simulink model "can8auto"  (R2018a)
settings: Solver=VariableStepAuto  StartTime=0.0  StopTime=5000  RelTol=1e-3
libraries: commcrc2 x20, simulink x20, simulink_extras x5, dspswit3 x5
(part 2 of 7)

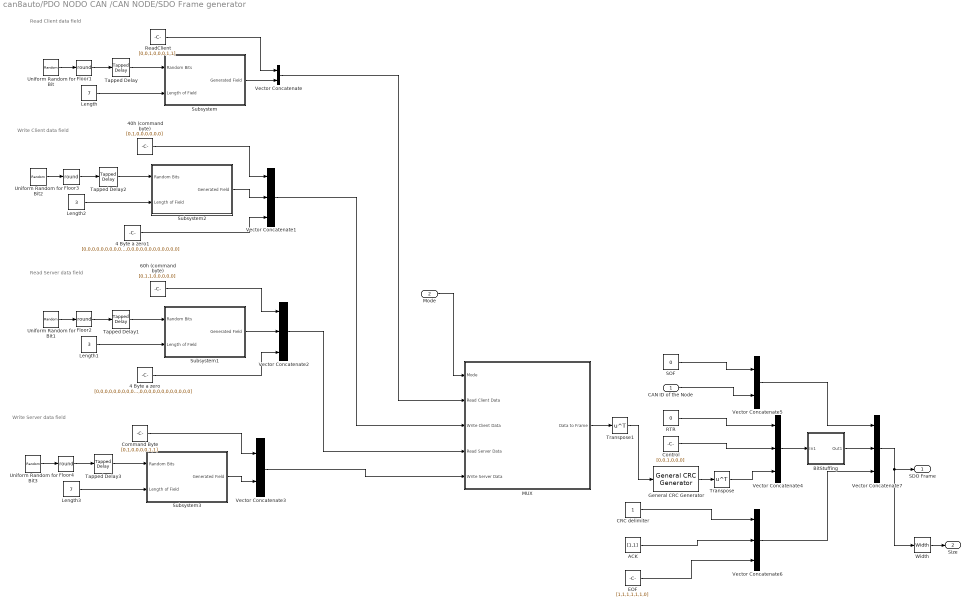
== system can8auto/PDO NODO CAN /CAN NODE/SDO Frame generator ==
  note: Read Server data field
  note: Read Client data field
  note: Write Client data field
  note: Write Server data field
  CAN ID of the Node : Inport
  Mode : Inport  Port=2
  4 Byte a zero : Constant  Value=[0,0,0,0,0,0,0,0,0,0,0,0,0,0,0,0,0,0,0,0,0,0,0,0,0,0,0,0,0,0,0,0]  VectorParams1D=off
  4 Byte a zero1 : Constant  Value=[0,0,0,0,0,0,0,0,0,0,0,0,0,0,0,0,0,0,0,0,0,0,0,0,0,0,0,0,0,0,0,0]  VectorParams1D=off
  40h (command byte) : Constant  Value=[0,1,0,0,0,0,0,0]  VectorParams1D=off
  60h (command byte) : Constant  Value=[0,1,1,0,0,0,0,0]  VectorParams1D=off
  ACK : Constant  Value=[1,1]  VectorParams1D=off
  BitStuffing : Subsystem
  CRC delimiter : Constant  VectorParams1D=off
  Command Byte : Constant  Value=[0,1,0,0,0,0,1,1]  VectorParams1D=off
  Control : Constant  Value=[0,0,1,0,0,0]  VectorParams1D=off
  EOF : Constant  Value=[1,1,1,1,1,1,0]  VectorParams1D=off
  Floor{1..4} (4 alike) : Rounding  Operator=round
  General CRC Generator : commcrc2/General CRC Generator  genPoly='z^15 + z^14 + z^10 + z^8 + z^7 + z^4 + z^3 + 1'  iniStates=0  directMethod=off  reflectInputBytes=off  reflectChecksums=off  finalXOR=0  numChecksums=1
      settings: SourceProductName=Communications Toolbox  SourceProductBaseCode=CM
  Length : Constant  Value=7  VectorParams1D=off
  Length1 : Constant  Value=3  VectorParams1D=off
  Length2 : Constant  Value=3  VectorParams1D=off
  Length3 : Constant  Value=7  VectorParams1D=off
  MUX : Subsystem
  RTR : Constant  Value=0  VectorParams1D=off
  ReadClient : Constant  Value=[0,0,1,0,0,0,1,1]  VectorParams1D=off
  SOF : Constant  Value=0  VectorParams1D=off
  Subsystem : Subsystem
  Subsystem1 : Subsystem
  Subsystem2 : Subsystem
  Subsystem3 : Subsystem
  Tapped Delay{,1..3} (4 alike) : simulink/Discrete/Tapped Delay  vinit=0  samptime=-1  NumDelays=8*8  DelayOrder=Oldest  includeCurrent=off
  Transpose : Math  Operator=transpose  SaturateOnIntegerOverflow=on
  Transpose1 : Math  Operator=transpose  SaturateOnIntegerOverflow=on
  Uniform Random for Bit{,1..3} (4 alike) : UniformRandomNumber  Minimum=0  SampleTime=0.01
  Vector Concatenate : Concatenate
  Vector Concatenate{1..2,4,6..7} (5 alike) : Concatenate  NumInputs=3
  Vector Concatenate3 : Concatenate
  Vector Concatenate5 : Concatenate
  Width : Width
  SDO Frame : Outport
  " Size" : Outport  Port=2
  wires:
  Vector Concatenate7/1 -> SDO Frame/1, Width/1
  Vector Concatenate5/1 -> Vector Concatenate7/1
  Vector Concatenate6/1 -> Vector Concatenate7/3
  BitStuffing/1(Out1) -> Vector Concatenate7/2
  Vector Concatenate4/1 -> BitStuffing/1(In1)
  RTR/1 -> Vector Concatenate4/1
  CRC delimiter/1 -> Vector Concatenate6/1
  ACK/1 -> Vector Concatenate6/2
  EOF/1 -> Vector Concatenate6/3
  CAN ID of the Node/1 -> Vector Concatenate5/2
  SOF/1 -> Vector Concatenate5/1
  MUX/1(Data to Frame) -> Transpose1/1
  Vector Concatenate3/1 -> MUX/5(Write Server Data)
  Vector Concatenate2/1 -> MUX/4(Read Server Data)
  Mode/1 -> MUX/1(Mode)
  Vector Concatenate1/1 -> MUX/3(Write Client Data)
  Vector Concatenate/1 -> MUX/2(Read Client Data)
  Width/1 -> " Size"/1
  ReadClient/1 -> Vector Concatenate/1
  Floor2/1 -> Tapped Delay1/1
  Subsystem/1(Generated Field) -> Vector Concatenate/2
  General CRC Generator/1 -> Transpose/1
  Length3/1 -> Subsystem3/2(Length of Field)
  Transpose/1 -> Vector Concatenate4/3
  4 Byte a zero/1 -> Vector Concatenate2/3
  4 Byte a zero1/1 -> Vector Concatenate1/3
  Control/1 -> Vector Concatenate4/2
  Subsystem2/1(Generated Field) -> Vector Concatenate1/2
  Tapped Delay1/1 -> Subsystem1/1(Random Bits)
  Floor1/1 -> Tapped Delay/1
  Uniform Random for Bit2/1 -> Floor3/1
  Subsystem1/1(Generated Field) -> Vector Concatenate2/2
  Subsystem3/1(Generated Field) -> Vector Concatenate3/2
  Command Byte/1 -> Vector Concatenate3/1
  Tapped Delay3/1 -> Subsystem3/1(Random Bits)
  Floor4/1 -> Tapped Delay3/1
  40h (command byte)/1 -> Vector Concatenate1/1
  Length2/1 -> Subsystem2/2(Length of Field)
  Uniform Random for Bit1/1 -> Floor2/1
  Length/1 -> Subsystem/2(Length of Field)
  Uniform Random for Bit3/1 -> Floor4/1
  Length1/1 -> Subsystem1/2(Length of Field)
  Tapped Delay/1 -> Subsystem/1(Random Bits)
  Floor3/1 -> Tapped Delay2/1
  Uniform Random for Bit/1 -> Floor1/1
  60h (command byte)/1 -> Vector Concatenate2/1
  Transpose1/1 -> General CRC Generator/1
  Tapped Delay2/1 -> Subsystem2/1(Random Bits)

== system can8auto/PDO NODO CAN /CAN NODE/SYNC Frame Generator ==
  ACK : Constant  Value=[1,1]  VectorParams1D=off
  BitStuffing : Subsystem
  COB ID (080h) : Constant  Value=[0,0,0,1,0,0,0,0,0,0,0]  VectorParams1D=off
  CRC delimiter : Constant  VectorParams1D=off
  Control : Constant  Value=[0,0,0,0,0,1]  VectorParams1D=off
  Data : Constant  Value=[0,0,0,0,0,0,0,0]'  VectorParams1D=off
  EOF : Constant  Value=[1,1,1,1,1,1,0]  VectorParams1D=off
  General CRC Generator : commcrc2/General CRC Generator  genPoly='z^15 + z^14 + z^10 + z^8 + z^7 + z^4 + z^3 + 1'  iniStates=0  directMethod=off  reflectInputBytes=off  reflectChecksums=off  finalXOR=0  numChecksums=1
      settings: SourceProductName=Communications Toolbox  SourceProductBaseCode=CM
  Mux1 : Mux  Inputs=3
  Mux2 : Mux  Inputs=2
  Mux3 : Mux  Inputs=3
  Mux4 : Mux  Inputs=3
  RTR : Constant  Value=0  VectorParams1D=off
  SOF : Constant  Value=0  VectorParams1D=off
  Transpose : Math  Operator=transpose  SaturateOnIntegerOverflow=on
  Width : Width
  SYNC Frame : Outport
  " Size" : Outport  Port=2
  wires:
  Mux4/1 -> SYNC Frame/1, Width/1
  Mux1/1 -> Mux4/1
  Mux2/1 -> Mux4/3
  BitStuffing/1(Out1) -> Mux4/2
  Mux3/1 -> BitStuffing/1(In1)
  Width/1 -> " Size"/1
  CRC delimiter/1 -> Mux3/3
  EOF/1 -> Mux2/2
  ACK/1 -> Mux2/1
  COB ID (080h)/1 -> Mux1/2
  SOF/1 -> Mux1/1
  Control/1 -> Mux3/1
  General CRC Generator/1 -> Transpose/1
  Transpose/1 -> Mux3/2
  RTR/1 -> Mux1/3
  Data/1 -> General CRC Generator/1

== system can8auto/PDO NODO CAN /CAN NODE/Triggered Subsystem1 ==
  In1 : Inport
  Trigger : TriggerPort  VariantControl=Variant
  Out1 : Outport  InitialOutput=[1,1,1,1,1,1,1,1,1,1,1,1,1,1,1,1,1,1,1,1,1,1,1,1,1,1,1,1,1,1,1,1,1,1,1,1,1,1,1,1,1,1,1,1,1,1,1,1,1,1,1,1,1,1,1,1,1,1,1,1,1,1,1,1,1,1,1,1,1,1,1,1,1,1,1,1,1,1,1,1,1,1,1,1]
  wires:
  In1/1 -> Out1/1

== system can8auto/PDO NODO CAN /Start on push/Start on push ==
  In1 : Inport
  Trigger : TriggerPort  VariantControl=Variant
  Out1 : Outport  InitialOutput=[0]
  wires:
  In1/1 -> Out1/1

== system can8auto/SDO NODO CAN/CAN NODE/Bootup Frame generator ==
  note: CAN ID / COB ID
  ID of the Node : Inport
  11-bit Adder : Subsystem
  700h : Constant  Value=[1,1,1,0,0,0,0,0,0,0,0]  VectorParams1D=off
  ACK : Constant  Value=[1,1]  VectorParams1D=off
  BitStuffing : Subsystem
  CRC delimiter : Constant  VectorParams1D=off
  Control : Constant  Value=[0,0,0,0,0,1]  VectorParams1D=off
  "Data (Bootup State) " : Constant  Value=[0,0,0,0,0,0,0,0]'  VectorParams1D=off
  EOF : Constant  Value=[1,1,1,1,1,1,0]  VectorParams1D=off
  General CRC Generator : commcrc2/General CRC Generator  genPoly='z^15 + z^14 + z^10 + z^8 + z^7 + z^4 + z^3 + 1'  iniStates=0  directMethod=off  reflectInputBytes=off  reflectChecksums=off  finalXOR=0  numChecksums=1
      settings: SourceProductName=Communications Toolbox  SourceProductBaseCode=CM
  Mux : Mux  Inputs=3
  Mux1 : Mux  Inputs=2
  Mux2 : Mux  Inputs=3
  Mux3 : Mux  Inputs=3
  RTR : Constant  Value=0  VectorParams1D=off
  SOF : Constant  Value=0  VectorParams1D=off
  Transpose : Math  Operator=transpose  SaturateOnIntegerOverflow=on
  Width : Width
  Bootload Frame : Outport
  " Size" : Outport  Port=2
  wires:
  Mux1/1 -> Mux3/1
  Mux2/1 -> Mux3/3
  BitStuffing/1(Out1) -> Mux3/2
  Mux3/1 -> Bootload Frame/1, Width/1
  Transpose/1 -> Mux/3
  RTR/1 -> Mux/1
  EOF/1 -> Mux2/3
  ACK/1 -> Mux2/2
  CRC delimiter/1 -> Mux2/1
  SOF/1 -> Mux1/1
  11-bit Adder/1(Out1) -> Mux1/2
  Width/1 -> " Size"/1
  ID of the Node/1 -> 11-bit Adder/2(In2)
  700h/1 -> 11-bit Adder/1(In1)
  Control/1 -> Mux/2
  "Data (Bootup State) "/1 -> General CRC Generator/1
  General CRC Generator/1 -> Transpose/1
  Mux/1 -> BitStuffing/1(In1)

== system can8auto/SDO NODO CAN/CAN NODE/Frame MUX ==
  Frame Kind : Inport
  Bootload Frame : Inport  Port=2
  Size Bootload : Inport  Port=3
  NMT Frame : Inport  Port=4
  Size NMT : Inport  Port=5
  SDO Frame : Inport  Port=6
  Size SDO : Inport  Port=7
  PDO Frame : Inport  Port=8
  Size PDO : Inport  Port=9
  SYNC Frame : Inport  Port=10
  Size SYNC : Inport  Port=11
  MATLAB Function2 : MATLAB Function  TreatAsAtomicUnit=on
  Vector Concatenate : Concatenate  NumInputs=5
  Vector Concatenate1 : Concatenate  NumInputs=5
  Frame to Send : Outport
  wires:
  Vector Concatenate1/1 -> MATLAB Function2/3(size)
  SYNC Frame/1 -> Vector Concatenate/5
  Size NMT/1 -> Vector Concatenate1/2
  Size SDO/1 -> Vector Concatenate1/3
  Size Bootload/1 -> Vector Concatenate1/1
  Size SYNC/1 -> Vector Concatenate1/5
  Vector Concatenate/1 -> MATLAB Function2/2(u1)
  SDO Frame/1 -> Vector Concatenate/3
  MATLAB Function2/1(result) -> Frame to Send/1
  Bootload Frame/1 -> Vector Concatenate/1
  PDO Frame/1 -> Vector Concatenate/4
  Frame Kind/1 -> MATLAB Function2/1(mode)
  NMT Frame/1 -> Vector Concatenate/2
  Size PDO/1 -> Vector Concatenate1/4

== system can8auto/SDO NODO CAN/CAN NODE/NMT Frame generator ==
  note: DATA FIELD
  Address node : Inport
  11-bit Adder : Subsystem
  ACK : Constant  Value=[1,1]  VectorParams1D=off
  BitStuffing : Subsystem
  COB ID : Constant  Value=[0,0,0,0,0,0,0,0,0,0,0]  VectorParams1D=off
  CRC delimiter : Constant  VectorParams1D=off
  Control : Constant  Value=[0,0,0,0,1,0]  VectorParams1D=off
  DATA (part1) : Constant  Value=[0,0,0,0,0]  VectorParams1D=off
  "Data " : Constant  Value=[0,0,1,0,0,0,0,0,0,0,0]  VectorParams1D=off
  EOF : Constant  Value=[1,1,1,1,1,1,0]  VectorParams1D=off
  General CRC Generator : commcrc2/General CRC Generator  genPoly='z^15 + z^14 + z^10 + z^8 + z^7 + z^4 + z^3 + 1'  iniStates=0  directMethod=off  reflectInputBytes=off  reflectChecksums=off  finalXOR=0  numChecksums=1
      settings: SourceProductName=Communications Toolbox  SourceProductBaseCode=CM
  Mux : Mux  Inputs=3
  Mux1 : Mux  Inputs=2
  Mux2 : Mux  Inputs=2
  Mux3 : Mux  Inputs=3
  Mux4 : Mux  Inputs=3
  RTR : Constant  Value=0  VectorParams1D=off
  SOF : Constant  Value=0  VectorParams1D=off
  Transpose : Math  Operator=transpose  SaturateOnIntegerOverflow=on
  Transpose1 : Math  Operator=transpose  SaturateOnIntegerOverflow=on
  Width : Width
  NMT Frame : Outport
  " Size" : Outport  Port=2
  wires:
  Mux4/1 -> Width/1, NMT Frame/1
  Mux3/1 -> Mux4/3
  Mux2/1 -> Mux4/1
  BitStuffing/1(Out1) -> Mux4/2
  Mux/1 -> BitStuffing/1(In1)
  RTR/1 -> Mux/1
  CRC delimiter/1 -> Mux3/1
  ACK/1 -> Mux3/2
  EOF/1 -> Mux3/3
  SOF/1 -> Mux2/1
  COB ID/1 -> Mux2/2
  Width/1 -> " Size"/1
  Transpose1/1 -> General CRC Generator/1
  Mux1/1 -> Transpose1/1
  11-bit Adder/1(Out1) -> Mux1/2
  DATA (part1)/1 -> Mux1/1
  "Data "/1 -> 11-bit Adder/1(In1)
  Address node/1 -> 11-bit Adder/2(In2)
  Transpose/1 -> Mux/3
  Control/1 -> Mux/2
  General CRC Generator/1 -> Transpose/1

== system can8auto/SDO NODO CAN/CAN NODE/PDO Frame Generator ==
  note: PDO DATA field
  note: CONTROL field
  CAN ID : Inport
  Data Length : Inport  Port=2
  " default = 8" : SwitchCase  CaseConditions={2,4}
  2 byte : Constant  Value=[0,0,0,0,1,0]  VectorParams1D=off
  4 byte : Constant  Value=[0,0,0,1,0,0]  VectorParams1D=off
  8 byte : Constant  Value=[0,0,1,0,0,0]  VectorParams1D=off
  ACK : Constant  Value=[1,1]  VectorParams1D=off
  CRC delimiter : Constant  VectorParams1D=off
  EOF : Constant  Value=[1,1,1,1,1,1,0]  VectorParams1D=off
  Floor1 : Rounding  Operator=round
  General CRC Generator : commcrc2/General CRC Generator  genPoly='z^15 + z^14 + z^10 + z^8 + z^7 + z^4 + z^3 + 1'  iniStates=0  directMethod=off  reflectInputBytes=off  reflectChecksums=off  finalXOR=0  numChecksums=1
      settings: SourceProductName=Communications Toolbox  SourceProductBaseCode=CM
  Merge1 : Merge  Inputs=3
  RTR : Constant  Value=0  VectorParams1D=off
  SOF : Constant  Value=0  VectorParams1D=off
  Subsystem : Subsystem
  Switch Case Action Subsystem : Subsystem  TreatAsAtomicUnit=on
  Switch Case Action Subsystem1 : Subsystem  TreatAsAtomicUnit=on
  Switch Case Action Subsystem2 : Subsystem  TreatAsAtomicUnit=on
  Tapped Delay : simulink/Discrete/Tapped Delay  vinit=0  samptime=-1  NumDelays=8*8  DelayOrder=Oldest  includeCurrent=off
  Uniform Random for Bit : UniformRandomNumber  Minimum=0  SampleTime=0.01
  Vector Concatenate1 : Concatenate  NumInputs=8
  Width : Width
  PDO Frame : Outport
  " Size" : Outport  Port=2
  wires:
  Vector Concatenate1/1 -> PDO Frame/1, Width/1
  Width/1 -> " Size"/1
  ACK/1 -> Vector Concatenate1/7
  EOF/1 -> Vector Concatenate1/8
  General CRC Generator/1 -> Vector Concatenate1/5
  Switch Case Action Subsystem1/1(Out1) -> Merge1/2
  2 byte/1 -> Switch Case Action Subsystem/1(In1)
  Tapped Delay/1 -> Subsystem/1(Random Bits)
  RTR/1 -> Vector Concatenate1/3
  Uniform Random for Bit/1 -> Floor1/1
  " default = 8"/3 -> Switch Case Action Subsystem2/Action
  Floor1/1 -> Tapped Delay/1
  SOF/1 -> Vector Concatenate1/1
  Data Length/1 -> " default = 8"/1, Subsystem/2(Length of Field)
  4 byte/1 -> Switch Case Action Subsystem1/1(In1)
  Subsystem/1(Generated Field) -> General CRC Generator/1
  " default = 8"/1 -> Switch Case Action Subsystem/Action
  CRC delimiter/1 -> Vector Concatenate1/6
  Merge1/1 -> Vector Concatenate1/4
  " default = 8"/2 -> Switch Case Action Subsystem1/Action
  8 byte/1 -> Switch Case Action Subsystem2/1(In1)
  CAN ID/1 -> Vector Concatenate1/2
  Switch Case Action Subsystem2/1(Out1) -> Merge1/3
  Switch Case Action Subsystem/1(Out1) -> Merge1/1

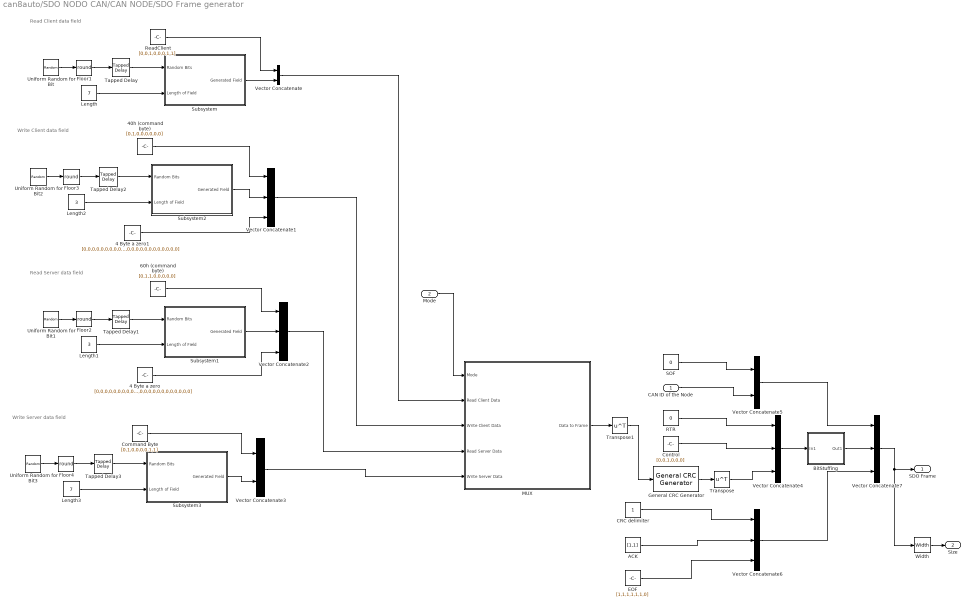
== system can8auto/SDO NODO CAN/CAN NODE/SDO Frame generator ==
  note: Read Server data field
  note: Read Client data field
  note: Write Client data field
  note: Write Server data field
  CAN ID of the Node : Inport
  Mode : Inport  Port=2
  4 Byte a zero : Constant  Value=[0,0,0,0,0,0,0,0,0,0,0,0,0,0,0,0,0,0,0,0,0,0,0,0,0,0,0,0,0,0,0,0]  VectorParams1D=off
  4 Byte a zero1 : Constant  Value=[0,0,0,0,0,0,0,0,0,0,0,0,0,0,0,0,0,0,0,0,0,0,0,0,0,0,0,0,0,0,0,0]  VectorParams1D=off
  40h (command byte) : Constant  Value=[0,1,0,0,0,0,0,0]  VectorParams1D=off
  60h (command byte) : Constant  Value=[0,1,1,0,0,0,0,0]  VectorParams1D=off
  ACK : Constant  Value=[1,1]  VectorParams1D=off
  BitStuffing : Subsystem
  CRC delimiter : Constant  VectorParams1D=off
  Command Byte : Constant  Value=[0,1,0,0,0,0,1,1]  VectorParams1D=off
  Control : Constant  Value=[0,0,1,0,0,0]  VectorParams1D=off
  EOF : Constant  Value=[1,1,1,1,1,1,0]  VectorParams1D=off
  Floor{1..4} (4 alike) : Rounding  Operator=round
  General CRC Generator : commcrc2/General CRC Generator  genPoly='z^15 + z^14 + z^10 + z^8 + z^7 + z^4 + z^3 + 1'  iniStates=0  directMethod=off  reflectInputBytes=off  reflectChecksums=off  finalXOR=0  numChecksums=1
      settings: SourceProductName=Communications Toolbox  SourceProductBaseCode=CM
  Length : Constant  Value=7  VectorParams1D=off
  Length1 : Constant  Value=3  VectorParams1D=off
  Length2 : Constant  Value=3  VectorParams1D=off
  Length3 : Constant  Value=7  VectorParams1D=off
  MUX : Subsystem
  RTR : Constant  Value=0  VectorParams1D=off
  ReadClient : Constant  Value=[0,0,1,0,0,0,1,1]  VectorParams1D=off
  SOF : Constant  Value=0  VectorParams1D=off
  Subsystem : Subsystem
  Subsystem1 : Subsystem
  Subsystem2 : Subsystem
  Subsystem3 : Subsystem
  Tapped Delay{,1..3} (4 alike) : simulink/Discrete/Tapped Delay  vinit=0  samptime=-1  NumDelays=8*8  DelayOrder=Oldest  includeCurrent=off
  Transpose : Math  Operator=transpose  SaturateOnIntegerOverflow=on
  Transpose1 : Math  Operator=transpose  SaturateOnIntegerOverflow=on
  Uniform Random for Bit{,1..3} (4 alike) : UniformRandomNumber  Minimum=0  SampleTime=0.01
  Vector Concatenate : Concatenate
  Vector Concatenate{1..2,4,6..7} (5 alike) : Concatenate  NumInputs=3
  Vector Concatenate3 : Concatenate
  Vector Concatenate5 : Concatenate
  Width : Width
  SDO Frame : Outport
  " Size" : Outport  Port=2
  wires:
  Vector Concatenate7/1 -> SDO Frame/1, Width/1
  Vector Concatenate5/1 -> Vector Concatenate7/1
  Vector Concatenate6/1 -> Vector Concatenate7/3
  BitStuffing/1(Out1) -> Vector Concatenate7/2
  Vector Concatenate4/1 -> BitStuffing/1(In1)
  RTR/1 -> Vector Concatenate4/1
  CRC delimiter/1 -> Vector Concatenate6/1
  ACK/1 -> Vector Concatenate6/2
  EOF/1 -> Vector Concatenate6/3
  CAN ID of the Node/1 -> Vector Concatenate5/2
  SOF/1 -> Vector Concatenate5/1
  MUX/1(Data to Frame) -> Transpose1/1
  Vector Concatenate3/1 -> MUX/5(Write Server Data)
  Vector Concatenate2/1 -> MUX/4(Read Server Data)
  Mode/1 -> MUX/1(Mode)
  Vector Concatenate1/1 -> MUX/3(Write Client Data)
  Vector Concatenate/1 -> MUX/2(Read Client Data)
  Width/1 -> " Size"/1
  ReadClient/1 -> Vector Concatenate/1
  Floor2/1 -> Tapped Delay1/1
  Subsystem/1(Generated Field) -> Vector Concatenate/2
  General CRC Generator/1 -> Transpose/1
  Length3/1 -> Subsystem3/2(Length of Field)
  Transpose/1 -> Vector Concatenate4/3
  4 Byte a zero/1 -> Vector Concatenate2/3
  4 Byte a zero1/1 -> Vector Concatenate1/3
  Control/1 -> Vector Concatenate4/2
  Subsystem2/1(Generated Field) -> Vector Concatenate1/2
  Tapped Delay1/1 -> Subsystem1/1(Random Bits)
  Floor1/1 -> Tapped Delay/1
  Uniform Random for Bit2/1 -> Floor3/1
  Subsystem1/1(Generated Field) -> Vector Concatenate2/2
  Subsystem3/1(Generated Field) -> Vector Concatenate3/2
  Command Byte/1 -> Vector Concatenate3/1
  Tapped Delay3/1 -> Subsystem3/1(Random Bits)
  Floor4/1 -> Tapped Delay3/1
  40h (command byte)/1 -> Vector Concatenate1/1
  Length2/1 -> Subsystem2/2(Length of Field)
  Uniform Random for Bit1/1 -> Floor2/1
  Length/1 -> Subsystem/2(Length of Field)
  Uniform Random for Bit3/1 -> Floor4/1
  Length1/1 -> Subsystem1/2(Length of Field)
  Tapped Delay/1 -> Subsystem/1(Random Bits)
  Floor3/1 -> Tapped Delay2/1
  Uniform Random for Bit/1 -> Floor1/1
  60h (command byte)/1 -> Vector Concatenate2/1
  Transpose1/1 -> General CRC Generator/1
  Tapped Delay2/1 -> Subsystem2/1(Random Bits)

== system can8auto/SDO NODO CAN/CAN NODE/SYNC Frame Generator ==
  ACK : Constant  Value=[1,1]  VectorParams1D=off
  BitStuffing : Subsystem
  COB ID (080h) : Constant  Value=[0,0,0,1,0,0,0,0,0,0,0]  VectorParams1D=off
  CRC delimiter : Constant  VectorParams1D=off
  Control : Constant  Value=[0,0,0,0,0,1]  VectorParams1D=off
  Data : Constant  Value=[0,0,0,0,0,0,0,0]'  VectorParams1D=off
  EOF : Constant  Value=[1,1,1,1,1,1,0]  VectorParams1D=off
  General CRC Generator : commcrc2/General CRC Generator  genPoly='z^15 + z^14 + z^10 + z^8 + z^7 + z^4 + z^3 + 1'  iniStates=0  directMethod=off  reflectInputBytes=off  reflectChecksums=off  finalXOR=0  numChecksums=1
      settings: SourceProductName=Communications Toolbox  SourceProductBaseCode=CM
  Mux1 : Mux  Inputs=3
  Mux2 : Mux  Inputs=2
  Mux3 : Mux  Inputs=3
  Mux4 : Mux  Inputs=3
  RTR : Constant  Value=0  VectorParams1D=off
  SOF : Constant  Value=0  VectorParams1D=off
  Transpose : Math  Operator=transpose  SaturateOnIntegerOverflow=on
  Width : Width
  SYNC Frame : Outport
  " Size" : Outport  Port=2
  wires:
  Mux4/1 -> SYNC Frame/1, Width/1
  Mux1/1 -> Mux4/1
  Mux2/1 -> Mux4/3
  BitStuffing/1(Out1) -> Mux4/2
  Mux3/1 -> BitStuffing/1(In1)
  Width/1 -> " Size"/1
  CRC delimiter/1 -> Mux3/3
  EOF/1 -> Mux2/2
  ACK/1 -> Mux2/1
  COB ID (080h)/1 -> Mux1/2
  SOF/1 -> Mux1/1
  Control/1 -> Mux3/1
  General CRC Generator/1 -> Transpose/1
  Transpose/1 -> Mux3/2
  RTR/1 -> Mux1/3
  Data/1 -> General CRC Generator/1

== system can8auto/SDO NODO CAN/CAN NODE/Triggered Subsystem1 ==
  In1 : Inport
  Trigger : TriggerPort  VariantControl=Variant
  Out1 : Outport  InitialOutput=[1]
  wires:
  In1/1 -> Out1/1

== system can8auto/SYNC PRODUCER/CAN NODE/Bootup Frame generator ==
  note: CAN ID / COB ID
  ID of the Node : Inport
  11-bit Adder : Subsystem
  700h : Constant  Value=[1,1,1,0,0,0,0,0,0,0,0]  VectorParams1D=off
  ACK : Constant  Value=[1,1]  VectorParams1D=off
  BitStuffing : Subsystem
  CRC delimiter : Constant  VectorParams1D=off
  Control : Constant  Value=[0,0,0,0,0,1]  VectorParams1D=off
  "Data (Bootup State) " : Constant  Value=[0,0,0,0,0,0,0,0]'  VectorParams1D=off
  EOF : Constant  Value=[1,1,1,1,1,1,0]  VectorParams1D=off
  General CRC Generator : commcrc2/General CRC Generator  genPoly='z^15 + z^14 + z^10 + z^8 + z^7 + z^4 + z^3 + 1'  iniStates=0  directMethod=off  reflectInputBytes=off  reflectChecksums=off  finalXOR=0  numChecksums=1
      settings: SourceProductName=Communications Toolbox  SourceProductBaseCode=CM
  Mux : Mux  Inputs=3
  Mux1 : Mux  Inputs=2
  Mux2 : Mux  Inputs=3
  Mux3 : Mux  Inputs=3
  RTR : Constant  Value=0  VectorParams1D=off
  SOF : Constant  Value=0  VectorParams1D=off
  Transpose : Math  Operator=transpose  SaturateOnIntegerOverflow=on
  Width : Width
  Bootload Frame : Outport
  " Size" : Outport  Port=2
  wires:
  Mux1/1 -> Mux3/1
  Mux2/1 -> Mux3/3
  BitStuffing/1(Out1) -> Mux3/2
  Mux3/1 -> Bootload Frame/1, Width/1
  Transpose/1 -> Mux/3
  RTR/1 -> Mux/1
  EOF/1 -> Mux2/3
  ACK/1 -> Mux2/2
  CRC delimiter/1 -> Mux2/1
  SOF/1 -> Mux1/1
  11-bit Adder/1(Out1) -> Mux1/2
  Width/1 -> " Size"/1
  ID of the Node/1 -> 11-bit Adder/2(In2)
  700h/1 -> 11-bit Adder/1(In1)
  Control/1 -> Mux/2
  "Data (Bootup State) "/1 -> General CRC Generator/1
  General CRC Generator/1 -> Transpose/1
  Mux/1 -> BitStuffing/1(In1)

== system can8auto/SYNC PRODUCER/CAN NODE/Frame MUX ==
  Frame Kind : Inport
  Bootload Frame : Inport  Port=2
  Size Bootload : Inport  Port=3
  NMT Frame : Inport  Port=4
  Size NMT : Inport  Port=5
  SDO Frame : Inport  Port=6
  Size SDO : Inport  Port=7
  PDO Frame : Inport  Port=8
  Size PDO : Inport  Port=9
  SYNC Frame : Inport  Port=10
  Size SYNC : Inport  Port=11
  MATLAB Function2 : MATLAB Function  TreatAsAtomicUnit=on
  Vector Concatenate : Concatenate  NumInputs=5
  Vector Concatenate1 : Concatenate  NumInputs=5
  Frame to Send : Outport
  wires:
  Vector Concatenate1/1 -> MATLAB Function2/3(size)
  SYNC Frame/1 -> Vector Concatenate/5
  Size NMT/1 -> Vector Concatenate1/2
  Size SDO/1 -> Vector Concatenate1/3
  Size Bootload/1 -> Vector Concatenate1/1
  Size SYNC/1 -> Vector Concatenate1/5
  Vector Concatenate/1 -> MATLAB Function2/2(u1)
  SDO Frame/1 -> Vector Concatenate/3
  MATLAB Function2/1(result) -> Frame to Send/1
  Bootload Frame/1 -> Vector Concatenate/1
  PDO Frame/1 -> Vector Concatenate/4
  Frame Kind/1 -> MATLAB Function2/1(mode)
  NMT Frame/1 -> Vector Concatenate/2
  Size PDO/1 -> Vector Concatenate1/4

== system can8auto/SYNC PRODUCER/CAN NODE/NMT Frame generator ==
  note: DATA FIELD
  Address node : Inport
  11-bit Adder : Subsystem
  ACK : Constant  Value=[1,1]  VectorParams1D=off
  BitStuffing : Subsystem
  COB ID : Constant  Value=[0,0,0,0,0,0,0,0,0,0,0]  VectorParams1D=off
  CRC delimiter : Constant  VectorParams1D=off
  Control : Constant  Value=[0,0,0,0,1,0]  VectorParams1D=off
  DATA (part1) : Constant  Value=[0,0,0,0,0]  VectorParams1D=off
  "Data " : Constant  Value=[0,0,1,0,0,0,0,0,0,0,0]  VectorParams1D=off
  EOF : Constant  Value=[1,1,1,1,1,1,0]  VectorParams1D=off
  General CRC Generator : commcrc2/General CRC Generator  genPoly='z^15 + z^14 + z^10 + z^8 + z^7 + z^4 + z^3 + 1'  iniStates=0  directMethod=off  reflectInputBytes=off  reflectChecksums=off  finalXOR=0  numChecksums=1
      settings: SourceProductName=Communications Toolbox  SourceProductBaseCode=CM
  Mux : Mux  Inputs=3
  Mux1 : Mux  Inputs=2
  Mux2 : Mux  Inputs=2
  Mux3 : Mux  Inputs=3
  Mux4 : Mux  Inputs=3
  RTR : Constant  Value=0  VectorParams1D=off
  SOF : Constant  Value=0  VectorParams1D=off
  Transpose : Math  Operator=transpose  SaturateOnIntegerOverflow=on
  Transpose1 : Math  Operator=transpose  SaturateOnIntegerOverflow=on
  Width : Width
  NMT Frame : Outport
  " Size" : Outport  Port=2
  wires:
  Mux4/1 -> Width/1, NMT Frame/1
  Mux3/1 -> Mux4/3
  Mux2/1 -> Mux4/1
  BitStuffing/1(Out1) -> Mux4/2
  Mux/1 -> BitStuffing/1(In1)
  RTR/1 -> Mux/1
  CRC delimiter/1 -> Mux3/1
  ACK/1 -> Mux3/2
  EOF/1 -> Mux3/3
  SOF/1 -> Mux2/1
  COB ID/1 -> Mux2/2
  Width/1 -> " Size"/1
  Transpose1/1 -> General CRC Generator/1
  Mux1/1 -> Transpose1/1
  11-bit Adder/1(Out1) -> Mux1/2
  DATA (part1)/1 -> Mux1/1
  "Data "/1 -> 11-bit Adder/1(In1)
  Address node/1 -> 11-bit Adder/2(In2)
  Transpose/1 -> Mux/3
  Control/1 -> Mux/2
  General CRC Generator/1 -> Transpose/1

== system can8auto/SYNC PRODUCER/CAN NODE/PDO Frame Generator ==
  note: PDO DATA field
  note: CONTROL field
  CAN ID : Inport
  Data Length : Inport  Port=2
  " default = 8" : SwitchCase  CaseConditions={2,4}
  2 byte : Constant  Value=[0,0,0,0,1,0]  VectorParams1D=off
  4 byte : Constant  Value=[0,0,0,1,0,0]  VectorParams1D=off
  8 byte : Constant  Value=[0,0,1,0,0,0]  VectorParams1D=off
  ACK : Constant  Value=[1,1]  VectorParams1D=off
  CRC delimiter : Constant  VectorParams1D=off
  EOF : Constant  Value=[1,1,1,1,1,1,0]  VectorParams1D=off
  Floor1 : Rounding  Operator=round
  General CRC Generator : commcrc2/General CRC Generator  genPoly='z^15 + z^14 + z^10 + z^8 + z^7 + z^4 + z^3 + 1'  iniStates=0  directMethod=off  reflectInputBytes=off  reflectChecksums=off  finalXOR=0  numChecksums=1
      settings: SourceProductName=Communications Toolbox  SourceProductBaseCode=CM
  Merge1 : Merge  Inputs=3
  RTR : Constant  Value=0  VectorParams1D=off
  SOF : Constant  Value=0  VectorParams1D=off
  Subsystem : Subsystem
  Switch Case Action Subsystem : Subsystem  TreatAsAtomicUnit=on
  Switch Case Action Subsystem1 : Subsystem  TreatAsAtomicUnit=on
  Switch Case Action Subsystem2 : Subsystem  TreatAsAtomicUnit=on
  Tapped Delay : simulink/Discrete/Tapped Delay  vinit=0  samptime=-1  NumDelays=8*8  DelayOrder=Oldest  includeCurrent=off
  Uniform Random for Bit : UniformRandomNumber  Minimum=0  SampleTime=0.01
  Vector Concatenate1 : Concatenate  NumInputs=8
  Width : Width
  PDO Frame : Outport
  " Size" : Outport  Port=2
  wires:
  Vector Concatenate1/1 -> PDO Frame/1, Width/1
  Width/1 -> " Size"/1
  ACK/1 -> Vector Concatenate1/7
  EOF/1 -> Vector Concatenate1/8
  General CRC Generator/1 -> Vector Concatenate1/5
  Switch Case Action Subsystem1/1(Out1) -> Merge1/2
  2 byte/1 -> Switch Case Action Subsystem/1(In1)
  Tapped Delay/1 -> Subsystem/1(Random Bits)
  RTR/1 -> Vector Concatenate1/3
  Uniform Random for Bit/1 -> Floor1/1
  " default = 8"/3 -> Switch Case Action Subsystem2/Action
  Floor1/1 -> Tapped Delay/1
  SOF/1 -> Vector Concatenate1/1
  Data Length/1 -> " default = 8"/1, Subsystem/2(Length of Field)
  4 byte/1 -> Switch Case Action Subsystem1/1(In1)
  Subsystem/1(Generated Field) -> General CRC Generator/1
  " default = 8"/1 -> Switch Case Action Subsystem/Action
  CRC delimiter/1 -> Vector Concatenate1/6
  Merge1/1 -> Vector Concatenate1/4
  " default = 8"/2 -> Switch Case Action Subsystem1/Action
  8 byte/1 -> Switch Case Action Subsystem2/1(In1)
  CAN ID/1 -> Vector Concatenate1/2
  Switch Case Action Subsystem2/1(Out1) -> Merge1/3
  Switch Case Action Subsystem/1(Out1) -> Merge1/1

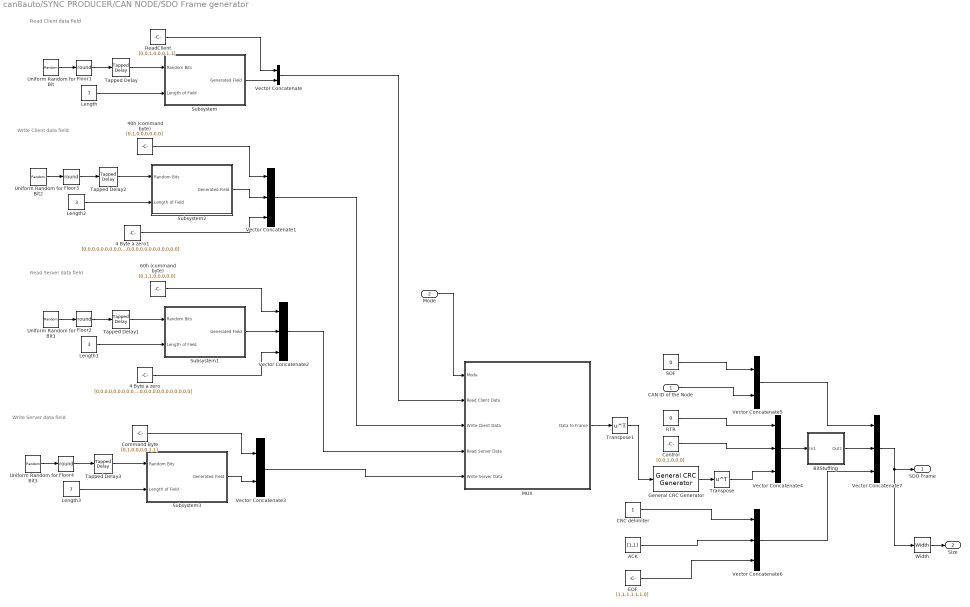
== system can8auto/SYNC PRODUCER/CAN NODE/SDO Frame generator ==
  note: Read Server data field
  note: Read Client data field
  note: Write Client data field
  note: Write Server data field
  CAN ID of the Node : Inport
  Mode : Inport  Port=2
  4 Byte a zero : Constant  Value=[0,0,0,0,0,0,0,0,0,0,0,0,0,0,0,0,0,0,0,0,0,0,0,0,0,0,0,0,0,0,0,0]  VectorParams1D=off
  4 Byte a zero1 : Constant  Value=[0,0,0,0,0,0,0,0,0,0,0,0,0,0,0,0,0,0,0,0,0,0,0,0,0,0,0,0,0,0,0,0]  VectorParams1D=off
  40h (command byte) : Constant  Value=[0,1,0,0,0,0,0,0]  VectorParams1D=off
  60h (command byte) : Constant  Value=[0,1,1,0,0,0,0,0]  VectorParams1D=off
  ACK : Constant  Value=[1,1]  VectorParams1D=off
  BitStuffing : Subsystem
  CRC delimiter : Constant  VectorParams1D=off
  Command Byte : Constant  Value=[0,1,0,0,0,0,1,1]  VectorParams1D=off
  Control : Constant  Value=[0,0,1,0,0,0]  VectorParams1D=off
  EOF : Constant  Value=[1,1,1,1,1,1,0]  VectorParams1D=off
  Floor{1..4} (4 alike) : Rounding  Operator=round
  General CRC Generator : commcrc2/General CRC Generator  genPoly='z^15 + z^14 + z^10 + z^8 + z^7 + z^4 + z^3 + 1'  iniStates=0  directMethod=off  reflectInputBytes=off  reflectChecksums=off  finalXOR=0  numChecksums=1
      settings: SourceProductName=Communications Toolbox  SourceProductBaseCode=CM
  Length : Constant  Value=7  VectorParams1D=off
  Length1 : Constant  Value=3  VectorParams1D=off
  Length2 : Constant  Value=3  VectorParams1D=off
  Length3 : Constant  Value=7  VectorParams1D=off
  MUX : Subsystem
  RTR : Constant  Value=0  VectorParams1D=off
  ReadClient : Constant  Value=[0,0,1,0,0,0,1,1]  VectorParams1D=off
  SOF : Constant  Value=0  VectorParams1D=off
  Subsystem : Subsystem
  Subsystem1 : Subsystem
  Subsystem2 : Subsystem
  Subsystem3 : Subsystem
  Tapped Delay{,1..3} (4 alike) : simulink/Discrete/Tapped Delay  vinit=0  samptime=-1  NumDelays=8*8  DelayOrder=Oldest  includeCurrent=off
  Transpose : Math  Operator=transpose  SaturateOnIntegerOverflow=on
  Transpose1 : Math  Operator=transpose  SaturateOnIntegerOverflow=on
  Uniform Random for Bit{,1..3} (4 alike) : UniformRandomNumber  Minimum=0  SampleTime=0.01
  Vector Concatenate : Concatenate
  Vector Concatenate{1..2,4,6..7} (5 alike) : Concatenate  NumInputs=3
  Vector Concatenate3 : Concatenate
  Vector Concatenate5 : Concatenate
  Width : Width
  SDO Frame : Outport
  " Size" : Outport  Port=2
  wires:
  Vector Concatenate7/1 -> SDO Frame/1, Width/1
  Vector Concatenate5/1 -> Vector Concatenate7/1
  Vector Concatenate6/1 -> Vector Concatenate7/3
  BitStuffing/1(Out1) -> Vector Concatenate7/2
  Vector Concatenate4/1 -> BitStuffing/1(In1)
  RTR/1 -> Vector Concatenate4/1
  CRC delimiter/1 -> Vector Concatenate6/1
  ACK/1 -> Vector Concatenate6/2
  EOF/1 -> Vector Concatenate6/3
  CAN ID of the Node/1 -> Vector Concatenate5/2
  SOF/1 -> Vector Concatenate5/1
  MUX/1(Data to Frame) -> Transpose1/1
  Vector Concatenate3/1 -> MUX/5(Write Server Data)
  Vector Concatenate2/1 -> MUX/4(Read Server Data)
  Mode/1 -> MUX/1(Mode)
  Vector Concatenate1/1 -> MUX/3(Write Client Data)
  Vector Concatenate/1 -> MUX/2(Read Client Data)
  Width/1 -> " Size"/1
  ReadClient/1 -> Vector Concatenate/1
  Floor2/1 -> Tapped Delay1/1
  Subsystem/1(Generated Field) -> Vector Concatenate/2
  General CRC Generator/1 -> Transpose/1
  Length3/1 -> Subsystem3/2(Length of Field)
  Transpose/1 -> Vector Concatenate4/3
  4 Byte a zero/1 -> Vector Concatenate2/3
  4 Byte a zero1/1 -> Vector Concatenate1/3
  Control/1 -> Vector Concatenate4/2
  Subsystem2/1(Generated Field) -> Vector Concatenate1/2
  Tapped Delay1/1 -> Subsystem1/1(Random Bits)
  Floor1/1 -> Tapped Delay/1
  Uniform Random for Bit2/1 -> Floor3/1
  Subsystem1/1(Generated Field) -> Vector Concatenate2/2
  Subsystem3/1(Generated Field) -> Vector Concatenate3/2
  Command Byte/1 -> Vector Concatenate3/1
  Tapped Delay3/1 -> Subsystem3/1(Random Bits)
  Floor4/1 -> Tapped Delay3/1
  40h (command byte)/1 -> Vector Concatenate1/1
  Length2/1 -> Subsystem2/2(Length of Field)
  Uniform Random for Bit1/1 -> Floor2/1
  Length/1 -> Subsystem/2(Length of Field)
  Uniform Random for Bit3/1 -> Floor4/1
  Length1/1 -> Subsystem1/2(Length of Field)
  Tapped Delay/1 -> Subsystem/1(Random Bits)
  Floor3/1 -> Tapped Delay2/1
  Uniform Random for Bit/1 -> Floor1/1
  60h (command byte)/1 -> Vector Concatenate2/1
  Transpose1/1 -> General CRC Generator/1
  Tapped Delay2/1 -> Subsystem2/1(Random Bits)

== system can8auto/SYNC PRODUCER/CAN NODE/SYNC Frame Generator ==
  ACK : Constant  Value=[1,1]  VectorParams1D=off
  BitStuffing : Subsystem
  COB ID (080h) : Constant  Value=[0,0,0,1,0,0,0,0,0,0,0]  VectorParams1D=off
  CRC delimiter : Constant  VectorParams1D=off
  Control : Constant  Value=[0,0,0,0,0,1]  VectorParams1D=off
  Data : Constant  Value=[0,0,0,0,0,0,0,0]'  VectorParams1D=off
  EOF : Constant  Value=[1,1,1,1,1,1,0]  VectorParams1D=off
  General CRC Generator : commcrc2/General CRC Generator  genPoly='z^15 + z^14 + z^10 + z^8 + z^7 + z^4 + z^3 + 1'  iniStates=0  directMethod=off  reflectInputBytes=off  reflectChecksums=off  finalXOR=0  numChecksums=1
      settings: SourceProductName=Communications Toolbox  SourceProductBaseCode=CM
  Mux1 : Mux  Inputs=3
  Mux2 : Mux  Inputs=2
  Mux3 : Mux  Inputs=3
  Mux4 : Mux  Inputs=3
  RTR : Constant  Value=0  VectorParams1D=off
  SOF : Constant  Value=0  VectorParams1D=off
  Transpose : Math  Operator=transpose  SaturateOnIntegerOverflow=on
  Width : Width
  SYNC Frame : Outport
  " Size" : Outport  Port=2
  wires:
  Mux4/1 -> SYNC Frame/1, Width/1
  Mux1/1 -> Mux4/1
  Mux2/1 -> Mux4/3
  BitStuffing/1(Out1) -> Mux4/2
  Mux3/1 -> BitStuffing/1(In1)
  Width/1 -> " Size"/1
  CRC delimiter/1 -> Mux3/3
  EOF/1 -> Mux2/2
  ACK/1 -> Mux2/1
  COB ID (080h)/1 -> Mux1/2
  SOF/1 -> Mux1/1
  Control/1 -> Mux3/1
  General CRC Generator/1 -> Transpose/1
  Transpose/1 -> Mux3/2
  RTR/1 -> Mux1/3
  Data/1 -> General CRC Generator/1

== system can8auto/SYNC PRODUCER/CAN NODE/Triggered Subsystem1 ==
  In1 : Inport
  Trigger : TriggerPort  VariantControl=Variant
  Out1 : Outport  InitialOutput=[1]
  wires:
  In1/1 -> Out1/1

== system can8auto/SYNC PRODUCER/Start on push/Start on push ==
  In1 : Inport
  Trigger : TriggerPort  VariantControl=Variant
  Out1 : Outport  InitialOutput=[0]
  wires:
  In1/1 -> Out1/1

== system can8auto/CAN MASTER/CAN NODE/Bootup Frame generator/11-bit Adder ==
  In1 : Inport
  In2 : Inport  Port=2
  8-bit Adder : Subsystem
  Data Type Conversion : DataTypeConversion
  Demux : Demux  Outputs=11
  Demux1 : Demux  Outputs=11
  Mux : Mux  Inputs=11
  Out1 : Outport
  wires:
  Data Type Conversion/1 -> Out1/1
  Mux/1 -> Data Type Conversion/1
  Demux1/11 -> 8-bit Adder/22(22)
  Demux1/10 -> 8-bit Adder/21(21)
  Demux1/9 -> 8-bit Adder/20(20)
  Demux1/8 -> 8-bit Adder/19(19)
  Demux1/7 -> 8-bit Adder/18(18)
  Demux1/6 -> 8-bit Adder/17(17)
  Demux1/5 -> 8-bit Adder/16(16)
  Demux1/4 -> 8-bit Adder/15(15)
  Demux1/3 -> 8-bit Adder/14(14)
  Demux1/2 -> 8-bit Adder/13(13)
  Demux1/1 -> 8-bit Adder/12(12)
  Demux/11 -> 8-bit Adder/11(11)
  Demux/10 -> 8-bit Adder/10(10)
  Demux/9 -> 8-bit Adder/9(9)
  Demux/8 -> 8-bit Adder/8(8)
  Demux/7 -> 8-bit Adder/7(7)
  Demux/6 -> 8-bit Adder/6(6)
  Demux/5 -> 8-bit Adder/5(5)
  Demux/4 -> 8-bit Adder/4(4)
  Demux/3 -> 8-bit Adder/3(3)
  Demux/2 -> 8-bit Adder/2(2)
  Demux/1 -> 8-bit Adder/1(1)
  8-bit Adder/11(out11) -> Mux/11
  8-bit Adder/10(out10) -> Mux/10
  8-bit Adder/9(out9) -> Mux/9
  8-bit Adder/8(out8) -> Mux/8
  8-bit Adder/7(out7) -> Mux/7
  8-bit Adder/6(out6) -> Mux/6
  8-bit Adder/5(out5) -> Mux/5
  8-bit Adder/4(out4) -> Mux/4
  8-bit Adder/3(out3) -> Mux/3
  8-bit Adder/2(out2) -> Mux/2
  8-bit Adder/1(out1) -> Mux/1
  In2/1 -> Demux1/1
  In1/1 -> Demux/1

== system can8auto/CAN MASTER/CAN NODE/Bootup Frame generator/BitStuffing ==
  In1 : Inport
  MATLAB Function : MATLAB Function  TreatAsAtomicUnit=on
  Out1 : Outport
  wires:
  In1/1 -> MATLAB Function/1(u)
  MATLAB Function/1(b) -> Out1/1

== system can8auto/CAN MASTER/CAN NODE/NMT Frame generator/11-bit Adder ==
  In1 : Inport
  In2 : Inport  Port=2
  11-bit Adder : Subsystem
  Data Type Conversion : DataTypeConversion
  Demux : Demux  Outputs=11
  Demux1 : Demux  Outputs=11
  Mux : Mux  Inputs=11
  Out1 : Outport
  wires:
  Data Type Conversion/1 -> Out1/1
  Demux1/11 -> 11-bit Adder/22(22)
  Demux1/10 -> 11-bit Adder/21(21)
  Demux1/9 -> 11-bit Adder/20(20)
  Demux1/8 -> 11-bit Adder/19(19)
  Demux1/7 -> 11-bit Adder/18(18)
  Demux1/6 -> 11-bit Adder/17(17)
  Demux1/5 -> 11-bit Adder/16(16)
  Demux1/4 -> 11-bit Adder/15(15)
  Demux1/3 -> 11-bit Adder/14(14)
  Demux1/2 -> 11-bit Adder/13(13)
  Demux1/1 -> 11-bit Adder/12(12)
  Demux/11 -> 11-bit Adder/11(11)
  Demux/10 -> 11-bit Adder/10(10)
  Demux/9 -> 11-bit Adder/9(9)
  Demux/8 -> 11-bit Adder/8(8)
  Demux/7 -> 11-bit Adder/7(7)
  Demux/6 -> 11-bit Adder/6(6)
  Demux/5 -> 11-bit Adder/5(5)
  Demux/4 -> 11-bit Adder/4(4)
  Demux/3 -> 11-bit Adder/3(3)
  Demux/2 -> 11-bit Adder/2(2)
  Demux/1 -> 11-bit Adder/1(1)
  11-bit Adder/11(out11) -> Mux/11
  11-bit Adder/10(out10) -> Mux/10
  11-bit Adder/9(out9) -> Mux/9
  11-bit Adder/8(out8) -> Mux/8
  11-bit Adder/7(out7) -> Mux/7
  11-bit Adder/6(out6) -> Mux/6
  11-bit Adder/5(out5) -> Mux/5
  11-bit Adder/4(out4) -> Mux/4
  11-bit Adder/3(out3) -> Mux/3
  11-bit Adder/2(out2) -> Mux/2
  11-bit Adder/1(out1) -> Mux/1
  In2/1 -> Demux1/1
  In1/1 -> Demux/1
  Mux/1 -> Data Type Conversion/1

== system can8auto/CAN MASTER/CAN NODE/NMT Frame generator/BitStuffing ==
  In1 : Inport
  MATLAB Function : MATLAB Function  TreatAsAtomicUnit=on
  Out1 : Outport
  wires:
  In1/1 -> MATLAB Function/1(u)
  MATLAB Function/1(b) -> Out1/1

== system can8auto/CAN MASTER/CAN NODE/PDO Frame Generator/Subsystem ==
  Random Bits : Inport
  Length of Field : Inport  Port=2
  1B : Subsystem  TreatAsAtomicUnit=on
  1B1 : Subsystem  TreatAsAtomicUnit=on
  1B2 : Subsystem  TreatAsAtomicUnit=on
  1B3 : Subsystem  TreatAsAtomicUnit=on
  1B4 : Subsystem  TreatAsAtomicUnit=on
  1B5 : Subsystem  TreatAsAtomicUnit=on
  1B6 : Subsystem  TreatAsAtomicUnit=on
  1B7 : Subsystem  TreatAsAtomicUnit=on
  Demux : Demux  Outputs=8
  Index Vector : MultiPortSwitch  Inputs=8  AllowDiffInputSizes=on
  Switch Case : SwitchCase  CaseConditions={1,2,3,4,5,6,7}
  Generated Field : Outport
  wires:
  Switch Case/8 -> 1B7/Action
  1B/1(Out1) -> Index Vector/2
  Demux/3 -> 1B2/3(In3), 1B6/3(In3), 1B4/3(In3), 1B3/3(In3), 1B7/3(In3), 1B5/3(In3)
  Random Bits/1 -> Demux/1
  Switch Case/3 -> 1B2/Action
  Switch Case/6 -> 1B5/Action
  Demux/2 -> 1B2/2(In2), 1B3/2(In2), 1B4/2(In2), 1B5/2(In2), 1B7/2(In2), 1B6/2(In2), 1B1/2(In2)
  1B2/1(Out1) -> Index Vector/4
  Switch Case/5 -> 1B4/Action
  1B3/1(Out1) -> Index Vector/5
  Demux/1 -> 1B1/1(In1), 1B/1(In1), 1B2/1(In1), 1B3/1(In1), 1B4/1(In1), 1B5/1(In1), 1B6/1(In1), 1B7/1(In1)
  Switch Case/2 -> 1B1/Action
  Switch Case/7 -> 1B6/Action
  Demux/4 -> 1B6/4(In4), 1B3/4(In4), 1B7/4(In4), 1B4/4(In4), 1B5/4(In4)
  1B1/1(Out1) -> Index Vector/3
  1B4/1(Out1) -> Index Vector/6
  Demux/8 -> 1B7/8(In8)
  Demux/7 -> 1B6/7(In7), 1B7/7(In7)
  Length of Field/1 -> Switch Case/1, Index Vector/1
  Switch Case/4 -> 1B3/Action
  Demux/5 -> 1B4/5(In5), 1B7/5(In5), 1B6/5(In5), 1B5/5(In5)
  Demux/6 -> 1B5/6(In6), 1B6/6(In6), 1B7/6(In6)
  1B6/1(Out1) -> Index Vector/8
  Switch Case/1 -> 1B/Action
  1B7/1(Out1) -> Index Vector/9
  1B5/1(Out1) -> Index Vector/7
  Index Vector/1 -> Generated Field/1

== system can8auto/CAN MASTER/CAN NODE/PDO Frame Generator/Switch Case Action Subsystem ==
  In1 : Inport
  Action Port : ActionPort  ActionType=case
  Out1 : Outport
  wires:
  In1/1 -> Out1/1

== system can8auto/CAN MASTER/CAN NODE/PDO Frame Generator/Switch Case Action Subsystem1 ==
  In1 : Inport
  Action Port : ActionPort  ActionType=case
  Out1 : Outport
  wires:
  In1/1 -> Out1/1

== system can8auto/CAN MASTER/CAN NODE/PDO Frame Generator/Switch Case Action Subsystem2 ==
  In1 : Inport
  Action Port : ActionPort  ActionType=default
  Out1 : Outport
  wires:
  In1/1 -> Out1/1

== system can8auto/CAN MASTER/CAN NODE/SDO Frame generator/BitStuffing ==
  In1 : Inport
  MATLAB Function : MATLAB Function  TreatAsAtomicUnit=on
  Out1 : Outport
  wires:
  In1/1 -> MATLAB Function/1(u)
  MATLAB Function/1(b) -> Out1/1

== system can8auto/CAN MASTER/CAN NODE/SDO Frame generator/MUX ==
  Mode : Inport
  Read Client Data : Inport  Port=2
  Write Client Data : Inport  Port=3
  Read Server Data : Inport  Port=4
  Write Server Data : Inport  Port=5
  Complex to Real-Imag : ComplexToRealImag  Output=Real
  MATLAB Function : MATLAB Function  TreatAsAtomicUnit=on
  Vector Concatenate5 : Concatenate  NumInputs=4
  Data to Frame : Outport
  wires:
  Read Server Data/1 -> Vector Concatenate5/3
  Complex to Real-Imag/1 -> Data to Frame/1
  MATLAB Function/1(result) -> Complex to Real-Imag/1
  Read Client Data/1 -> Vector Concatenate5/1
  Vector Concatenate5/1 -> MATLAB Function/2(u1)
  Write Server Data/1 -> Vector Concatenate5/4
  Mode/1 -> MATLAB Function/1(index)
  Write Client Data/1 -> Vector Concatenate5/2

== system can8auto/CAN MASTER/CAN NODE/SDO Frame generator/Subsystem ==
  Random Bits : Inport
  Length of Field : Inport  Port=2
  1B : Subsystem  TreatAsAtomicUnit=on
  1B1 : Subsystem  TreatAsAtomicUnit=on
  1B2 : Subsystem  TreatAsAtomicUnit=on
  1B3 : Subsystem  TreatAsAtomicUnit=on
  1B4 : Subsystem  TreatAsAtomicUnit=on
  1B5 : Subsystem  TreatAsAtomicUnit=on
  1B6 : Subsystem  TreatAsAtomicUnit=on
  1B7 : Subsystem  TreatAsAtomicUnit=on
  Demux : Demux  Outputs=8
  Index Vector : MultiPortSwitch  Inputs=8  AllowDiffInputSizes=on
  Switch Case : SwitchCase  CaseConditions={1,2,3,4,5,6,7}
  Generated Field : Outport
  wires:
  Switch Case/8 -> 1B7/Action
  1B/1(Out1) -> Index Vector/2
  Demux/3 -> 1B2/3(In3), 1B6/3(In3), 1B4/3(In3), 1B3/3(In3), 1B7/3(In3), 1B5/3(In3)
  Random Bits/1 -> Demux/1
  Switch Case/3 -> 1B2/Action
  Switch Case/6 -> 1B5/Action
  Demux/2 -> 1B2/2(In2), 1B3/2(In2), 1B4/2(In2), 1B5/2(In2), 1B7/2(In2), 1B6/2(In2), 1B1/2(In2)
  1B2/1(Out1) -> Index Vector/4
  Switch Case/5 -> 1B4/Action
  1B3/1(Out1) -> Index Vector/5
  Demux/1 -> 1B1/1(In1), 1B/1(In1), 1B2/1(In1), 1B3/1(In1), 1B4/1(In1), 1B5/1(In1), 1B6/1(In1), 1B7/1(In1)
  Switch Case/2 -> 1B1/Action
  Switch Case/7 -> 1B6/Action
  Demux/4 -> 1B6/4(In4), 1B3/4(In4), 1B7/4(In4), 1B4/4(In4), 1B5/4(In4)
  1B1/1(Out1) -> Index Vector/3
  1B4/1(Out1) -> Index Vector/6
  Demux/8 -> 1B7/8(In8)
  Demux/7 -> 1B6/7(In7), 1B7/7(In7)
  Length of Field/1 -> Switch Case/1, Index Vector/1
  Switch Case/4 -> 1B3/Action
  Demux/5 -> 1B4/5(In5), 1B7/5(In5), 1B6/5(In5), 1B5/5(In5)
  Demux/6 -> 1B5/6(In6), 1B6/6(In6), 1B7/6(In6)
  1B6/1(Out1) -> Index Vector/8
  Switch Case/1 -> 1B/Action
  1B7/1(Out1) -> Index Vector/9
  1B5/1(Out1) -> Index Vector/7
  Index Vector/1 -> Generated Field/1

== system can8auto/CAN MASTER/CAN NODE/SDO Frame generator/Subsystem1 ==
  Random Bits : Inport
  Length of Field : Inport  Port=2
  1B : Subsystem  TreatAsAtomicUnit=on
  1B1 : Subsystem  TreatAsAtomicUnit=on
  1B2 : Subsystem  TreatAsAtomicUnit=on
  1B3 : Subsystem  TreatAsAtomicUnit=on
  1B4 : Subsystem  TreatAsAtomicUnit=on
  1B5 : Subsystem  TreatAsAtomicUnit=on
  1B6 : Subsystem  TreatAsAtomicUnit=on
  1B7 : Subsystem  TreatAsAtomicUnit=on
  Demux : Demux  Outputs=8
  Index Vector : MultiPortSwitch  Inputs=8  AllowDiffInputSizes=on
  Switch Case : SwitchCase  CaseConditions={1,2,3,4,5,6,7}
  Generated Field : Outport
  wires:
  Switch Case/8 -> 1B7/Action
  1B/1(Out1) -> Index Vector/2
  Demux/3 -> 1B2/3(In3), 1B6/3(In3), 1B4/3(In3), 1B3/3(In3), 1B7/3(In3), 1B5/3(In3)
  Random Bits/1 -> Demux/1
  Switch Case/3 -> 1B2/Action
  Switch Case/6 -> 1B5/Action
  Demux/2 -> 1B2/2(In2), 1B3/2(In2), 1B4/2(In2), 1B5/2(In2), 1B7/2(In2), 1B6/2(In2), 1B1/2(In2)
  1B2/1(Out1) -> Index Vector/4
  Switch Case/5 -> 1B4/Action
  1B3/1(Out1) -> Index Vector/5
  Demux/1 -> 1B1/1(In1), 1B/1(In1), 1B2/1(In1), 1B3/1(In1), 1B4/1(In1), 1B5/1(In1), 1B6/1(In1), 1B7/1(In1)
  Switch Case/2 -> 1B1/Action
  Switch Case/7 -> 1B6/Action
  Demux/4 -> 1B6/4(In4), 1B3/4(In4), 1B7/4(In4), 1B4/4(In4), 1B5/4(In4)
  1B1/1(Out1) -> Index Vector/3
  1B4/1(Out1) -> Index Vector/6
  Demux/8 -> 1B7/8(In8)
  Demux/7 -> 1B6/7(In7), 1B7/7(In7)
  Length of Field/1 -> Index Vector/1, Switch Case/1
  Switch Case/4 -> 1B3/Action
  Demux/5 -> 1B4/5(In5), 1B7/5(In5), 1B6/5(In5), 1B5/5(In5)
  Demux/6 -> 1B5/6(In6), 1B6/6(In6), 1B7/6(In6)
  1B6/1(Out1) -> Index Vector/8
  Switch Case/1 -> 1B/Action
  1B7/1(Out1) -> Index Vector/9
  1B5/1(Out1) -> Index Vector/7
  Index Vector/1 -> Generated Field/1

== system can8auto/CAN MASTER/CAN NODE/SDO Frame generator/Subsystem2 ==
  Random Bits : Inport
  Length of Field : Inport  Port=2
  1B : Subsystem  TreatAsAtomicUnit=on
  1B1 : Subsystem  TreatAsAtomicUnit=on
  1B2 : Subsystem  TreatAsAtomicUnit=on
  1B3 : Subsystem  TreatAsAtomicUnit=on
  1B4 : Subsystem  TreatAsAtomicUnit=on
  1B5 : Subsystem  TreatAsAtomicUnit=on
  1B6 : Subsystem  TreatAsAtomicUnit=on
  1B7 : Subsystem  TreatAsAtomicUnit=on
  Demux : Demux  Outputs=8
  Index Vector : MultiPortSwitch  Inputs=8  AllowDiffInputSizes=on
  Switch Case : SwitchCase  CaseConditions={1,2,3,4,5,6,7}
  Generated Field : Outport
  wires:
  Switch Case/8 -> 1B7/Action
  1B/1(Out1) -> Index Vector/2
  Demux/3 -> 1B2/3(In3), 1B6/3(In3), 1B4/3(In3), 1B3/3(In3), 1B7/3(In3), 1B5/3(In3)
  Random Bits/1 -> Demux/1
  Switch Case/3 -> 1B2/Action
  Switch Case/6 -> 1B5/Action
  Demux/2 -> 1B2/2(In2), 1B3/2(In2), 1B4/2(In2), 1B5/2(In2), 1B7/2(In2), 1B6/2(In2), 1B1/2(In2)
  1B2/1(Out1) -> Index Vector/4
  Switch Case/5 -> 1B4/Action
  1B3/1(Out1) -> Index Vector/5
  Demux/1 -> 1B1/1(In1), 1B/1(In1), 1B2/1(In1), 1B3/1(In1), 1B4/1(In1), 1B5/1(In1), 1B6/1(In1), 1B7/1(In1)
  Switch Case/2 -> 1B1/Action
  Switch Case/7 -> 1B6/Action
  Demux/4 -> 1B6/4(In4), 1B3/4(In4), 1B7/4(In4), 1B4/4(In4), 1B5/4(In4)
  1B1/1(Out1) -> Index Vector/3
  1B4/1(Out1) -> Index Vector/6
  Demux/8 -> 1B7/8(In8)
  Demux/7 -> 1B6/7(In7), 1B7/7(In7)
  Length of Field/1 -> Switch Case/1, Index Vector/1
  Switch Case/4 -> 1B3/Action
  Demux/5 -> 1B4/5(In5), 1B7/5(In5), 1B6/5(In5), 1B5/5(In5)
  Demux/6 -> 1B5/6(In6), 1B6/6(In6), 1B7/6(In6)
  1B6/1(Out1) -> Index Vector/8
  Switch Case/1 -> 1B/Action
  1B7/1(Out1) -> Index Vector/9
  1B5/1(Out1) -> Index Vector/7
  Index Vector/1 -> Generated Field/1

== system can8auto/CAN MASTER/CAN NODE/SDO Frame generator/Subsystem3 ==
  Random Bits : Inport
  Length of Field : Inport  Port=2
  1B : Subsystem  TreatAsAtomicUnit=on
  1B1 : Subsystem  TreatAsAtomicUnit=on
  1B2 : Subsystem  TreatAsAtomicUnit=on
  1B3 : Subsystem  TreatAsAtomicUnit=on
  1B4 : Subsystem  TreatAsAtomicUnit=on
  1B5 : Subsystem  TreatAsAtomicUnit=on
  1B6 : Subsystem  TreatAsAtomicUnit=on
  1B7 : Subsystem  TreatAsAtomicUnit=on
  Demux : Demux  Outputs=8
  Index Vector : MultiPortSwitch  Inputs=8  AllowDiffInputSizes=on
  Switch Case : SwitchCase  CaseConditions={1,2,3,4,5,6,7}
  Generated Field : Outport
  wires:
  Switch Case/8 -> 1B7/Action
  1B/1(Out1) -> Index Vector/2
  Demux/3 -> 1B2/3(In3), 1B6/3(In3), 1B4/3(In3), 1B3/3(In3), 1B7/3(In3), 1B5/3(In3)
  Random Bits/1 -> Demux/1
  Switch Case/3 -> 1B2/Action
  Switch Case/6 -> 1B5/Action
  Demux/2 -> 1B2/2(In2), 1B3/2(In2), 1B4/2(In2), 1B5/2(In2), 1B7/2(In2), 1B6/2(In2), 1B1/2(In2)
  1B2/1(Out1) -> Index Vector/4
  Switch Case/5 -> 1B4/Action
  1B3/1(Out1) -> Index Vector/5
  Demux/1 -> 1B1/1(In1), 1B/1(In1), 1B2/1(In1), 1B3/1(In1), 1B4/1(In1), 1B5/1(In1), 1B6/1(In1), 1B7/1(In1)
  Switch Case/2 -> 1B1/Action
  Switch Case/7 -> 1B6/Action
  Demux/4 -> 1B6/4(In4), 1B3/4(In4), 1B7/4(In4), 1B4/4(In4), 1B5/4(In4)
  1B1/1(Out1) -> Index Vector/3
  1B4/1(Out1) -> Index Vector/6
  Demux/8 -> 1B7/8(In8)
  Demux/7 -> 1B6/7(In7), 1B7/7(In7)
  Length of Field/1 -> Switch Case/1, Index Vector/1
  Switch Case/4 -> 1B3/Action
  Demux/5 -> 1B4/5(In5), 1B7/5(In5), 1B6/5(In5), 1B5/5(In5)
  Demux/6 -> 1B5/6(In6), 1B6/6(In6), 1B7/6(In6)
  1B6/1(Out1) -> Index Vector/8
  Switch Case/1 -> 1B/Action
  1B7/1(Out1) -> Index Vector/9
  1B5/1(Out1) -> Index Vector/7
  Index Vector/1 -> Generated Field/1

== system can8auto/CAN MASTER/CAN NODE/SYNC Frame Generator/BitStuffing ==
  In1 : Inport
  MATLAB Function : MATLAB Function  TreatAsAtomicUnit=on
  Out1 : Outport
  wires:
  In1/1 -> MATLAB Function/1(u)
  MATLAB Function/1(b) -> Out1/1

== system can8auto/PDO NODO CAN /CAN NODE/Bootup Frame generator/11-bit Adder ==
  In1 : Inport
  In2 : Inport  Port=2
  8-bit Adder : Subsystem
  Data Type Conversion : DataTypeConversion
  Demux : Demux  Outputs=11
  Demux1 : Demux  Outputs=11
  Mux : Mux  Inputs=11
  Out1 : Outport
  wires:
  Data Type Conversion/1 -> Out1/1
  Mux/1 -> Data Type Conversion/1
  Demux1/11 -> 8-bit Adder/22(22)
  Demux1/10 -> 8-bit Adder/21(21)
  Demux1/9 -> 8-bit Adder/20(20)
  Demux1/8 -> 8-bit Adder/19(19)
  Demux1/7 -> 8-bit Adder/18(18)
  Demux1/6 -> 8-bit Adder/17(17)
  Demux1/5 -> 8-bit Adder/16(16)
  Demux1/4 -> 8-bit Adder/15(15)
  Demux1/3 -> 8-bit Adder/14(14)
  Demux1/2 -> 8-bit Adder/13(13)
  Demux1/1 -> 8-bit Adder/12(12)
  Demux/11 -> 8-bit Adder/11(11)
  Demux/10 -> 8-bit Adder/10(10)
  Demux/9 -> 8-bit Adder/9(9)
  Demux/8 -> 8-bit Adder/8(8)
  Demux/7 -> 8-bit Adder/7(7)
  Demux/6 -> 8-bit Adder/6(6)
  Demux/5 -> 8-bit Adder/5(5)
  Demux/4 -> 8-bit Adder/4(4)
  Demux/3 -> 8-bit Adder/3(3)
  Demux/2 -> 8-bit Adder/2(2)
  Demux/1 -> 8-bit Adder/1(1)
  8-bit Adder/11(out11) -> Mux/11
  8-bit Adder/10(out10) -> Mux/10
  8-bit Adder/9(out9) -> Mux/9
  8-bit Adder/8(out8) -> Mux/8
  8-bit Adder/7(out7) -> Mux/7
  8-bit Adder/6(out6) -> Mux/6
  8-bit Adder/5(out5) -> Mux/5
  8-bit Adder/4(out4) -> Mux/4
  8-bit Adder/3(out3) -> Mux/3
  8-bit Adder/2(out2) -> Mux/2
  8-bit Adder/1(out1) -> Mux/1
  In2/1 -> Demux1/1
  In1/1 -> Demux/1

== system can8auto/PDO NODO CAN /CAN NODE/Bootup Frame generator/BitStuffing ==
  In1 : Inport
  MATLAB Function : MATLAB Function  TreatAsAtomicUnit=on
  Out1 : Outport
  wires:
  In1/1 -> MATLAB Function/1(u)
  MATLAB Function/1(b) -> Out1/1
